simulink model "Boeing787_NewMission_ElectricalThermal_2013"  (R2013a)
settings: Solver=ode23tb  SolverMode=SingleTasking  StartTime=0.0  StopTime=18000  RelTol=1e-3
InitFcn:
  | load('SampleOutput.mat')
  | 
  | load('SampleFuelBurn.mat')
StartFcn:
  | tic
StopFcn:
  | ttt = toc
  | tend = eval(get_param(bdroot,'StopTime'));
  | disp(['Total Simulation Time (s) = ' num2str(ttt) 's']);
  | RTR =  ttt/tend
  | disp(['Simulation Speed is ' num2str(tend/ttt) 'x faster than real-time']);
values from neighbouring files (symbols this model uses):
  CurrentMission = Mission(i)    [mission_plan.m]
  seed = 1    [mission_plan.m]
undefined symbols (not defined in the file or in its folder): FuelBurn
libraries: PowerFlowLib x17, simulink x12, powerlib_meascontrol x1
(part 14 of 17)

== system Boeing787_NewMission_ElectricalThermal_2013/Eng2/Gearbox ==
  w_engine : Inport
  T_gen : Inport  Port=2
  1-tran_efficiency : Gain  Gain=1-Gear_Efficiency/100  SaturateOnIntegerOverflow=on  OutDataTypeStr=Inherit: Same as input  ParamDataTypeStr=Inherit: Same as input
  Gain : Gain  Gain=Gear_Ratio
  Gain1 : Gain  Gain=Gear_Ratio
  Memory1 : Memory
  Sum : Sum  Inputs=-++  SaturateOnIntegerOverflow=on  InputSameDT=on  OutDataTypeStr=Inherit: Same as first input
  gear1 NL loss : Lookup  InputValues=[0;1000;2000;3000;4000;5000;6000]*2*pi/60  Table=[0;0.735;1.334;1.491;1.525;1.212;1.276]  SaturateOnIntegerOverflow=on
  tran_efficiency : Gain  Gain=Gear_Efficiency/4/100  SaturateOnIntegerOverflow=on  OutDataTypeStr=Inherit: Same as input  ParamDataTypeStr=Inherit: Same as input
  w_shaft : Outport
  T_shaft : Outport  Port=2
  wires:
  Sum/1 -> T_shaft/1
  tran_efficiency/1 -> Sum/1
  1-tran_efficiency/1 -> Sum/2
  Memory1/1 -> Sum/3
  gear1 NL loss/1 -> tran_efficiency/1
  w_engine/1 -> gear1 NL loss/1, Gain/1
  T_gen/1 -> 1-tran_efficiency/1, Gain1/1
  Gain1/1 -> Memory1/1
  Gain/1 -> w_shaft/1

== system Boeing787_NewMission_ElectricalThermal_2013/Eng2/Unit Conversion  ==
  Signal_in : Inport
  conv_fcn : Fcn  Expr=u(1)/745.69987
  Converted Signal Out : Outport
  wires:
  conv_fcn/1 -> Converted Signal Out/1
  Signal_in/1 -> conv_fcn/1

== system Boeing787_NewMission_ElectricalThermal_2013/Eng2/Unit Conversion 1 ==
  Signal_in : Inport
  conv_fcn : Fcn  Expr=u(1)/1.8
  Converted Signal Out : Outport
  wires:
  Signal_in/1 -> conv_fcn/1
  conv_fcn/1 -> Converted Signal Out/1

== system Boeing787_NewMission_ElectricalThermal_2013/Eng2/Unit Conversion 4 ==
  Signal_in : Inport
  conv_fcn : Fcn  Expr=u(1)/(1.450377e-1)
  Converted Signal Out : Outport
  wires:
  conv_fcn/1 -> Converted Signal Out/1
  Signal_in/1 -> conv_fcn/1

== system Boeing787_NewMission_ElectricalThermal_2013/Eng2/Unit Conversion 5 ==
  Signal_in : Inport
  conv_fcn : Fcn  Expr=u(1)*.45359237
  Converted Signal Out : Outport
  wires:
  conv_fcn/1 -> Converted Signal Out/1
  Signal_in/1 -> conv_fcn/1

== system Boeing787_NewMission_ElectricalThermal_2013/Electrical/Auto Transformer/Control ==
  Vout : Inport
  ref : Inport  Port=2
  Clock : Clock
  Constant2 : Constant  Value=0
  Integrator : Integrator  ExternalReset=rising
  MinMax : MinMax  Function=max
  Reset on controller start : Step  Time=75  SampleTime=0
  Sum : Sum  Inputs=|-+
  Switch : Switch  Criteria=u2 > Threshold  Threshold=75
  u : Outport
  wires:
  Integrator/1 -> Switch/1
  Vout/1 -> MinMax/1
  Reset on controller start/1 -> Integrator/2
  Switch/1 -> u/1
  Constant2/1 -> Switch/3
  Clock/1 -> Switch/2
  ref/1 -> Sum/2
  Sum/1 -> Integrator/1
  MinMax/1 -> Sum/1

== system Boeing787_NewMission_ElectricalThermal_2013/Electrical/Auto Transformer/Transformer1 ==
  Vin : Inport
  Iout : Inport  Port=2
  u : Inport  Port=3
  Constant : Constant  Value=N2/N1
  Constant1 : Constant  Value=N2/N1
  Gain2 : Gain  Gain=Rp
  Gain3 : Gain  Gain=Rs
  Product : Product  Inputs=3
  Product1 : Product  Inputs=3
  Sum1 : Sum  Inputs=|+-
  Sum2 : Sum  Inputs=|+-
  Vout : Outport
  Iin : Outport  Port=2
  wires:
  Iout/1 -> Product1/3, Gain3/1
  Vin/1 -> Sum1/1
  Gain2/1 -> Sum1/2
  Sum1/1 -> Product/2
  Sum2/1 -> Vout/1
  Gain3/1 -> Sum2/2
  u/1 -> Product1/1, Product/1
  Product/1 -> Sum2/1
  Constant/1 -> Product/3
  Constant1/1 -> Product1/2
  Product1/1 -> Gain2/1, Iin/1

== system Boeing787_NewMission_ElectricalThermal_2013/Electrical/Enabled_AC_Loadloss/Enabled Subsystem ==
  "Vdq0 " : Inport
  CURRENT BASED LOADS : Subsystem
  IMPEDANCE BASED LOADS : Subsystem
  POWER BASED LOADS : Subsystem
  Sum of Elements : Sum  Inputs=+++
  Idq0 : Outport
  loss : Outport  Port=2
  wires:
  POWER BASED LOADS/2(loss) -> loss/1
  IMPEDANCE BASED LOADS/1(Idq0) -> Sum of Elements/3
  Sum of Elements/1 -> Idq0/1
  CURRENT BASED LOADS/1(Idqo) -> Sum of Elements/2
  POWER BASED LOADS/1(Idq0) -> Sum of Elements/1
  "Vdq0 "/1 -> POWER BASED LOADS/1(Vdq0), IMPEDANCE BASED LOADS/1(Vdq0)

== system Boeing787_NewMission_ElectricalThermal_2013/Electrical/Enabled_AC_Loadloss/Enabled Subsystem1 ==
  "Vdq0 " : Inport
  Ext vector : Inport  Port=2
  CURRENT BASED LOADS : Subsystem
  Demux : Demux  Outputs=3
  POWER BASED LOADS : Subsystem
  Sum of Elements : Sum
  Idq0 : Outport
  wires:
  Demux/3 -> CURRENT BASED LOADS/1(Iconst RMS)
  Demux/2 -> POWER BASED LOADS/3(Q)
  Demux/1 -> POWER BASED LOADS/2(P)
  "Vdq0 "/1 -> POWER BASED LOADS/1(Vdq0)
  Ext vector/1 -> Demux/1
  Sum of Elements/1 -> Idq0/1
  POWER BASED LOADS/1(Idq0) -> Sum of Elements/1
  CURRENT BASED LOADS/1(Idqo) -> Sum of Elements/2

== system Boeing787_NewMission_ElectricalThermal_2013/Electrical/Enabled_AC_Loadloss1/Enabled Subsystem ==
  "Vdq0 " : Inport
  CURRENT BASED LOADS : Subsystem
  IMPEDANCE BASED LOADS : Subsystem
  POWER BASED LOADS : Subsystem
  Sum of Elements : Sum  Inputs=+++
  Idq0 : Outport
  loss : Outport  Port=2
  wires:
  POWER BASED LOADS/2(loss) -> loss/1
  IMPEDANCE BASED LOADS/1(Idq0) -> Sum of Elements/3
  CURRENT BASED LOADS/1(Idqo) -> Sum of Elements/2
  POWER BASED LOADS/1(Idq0) -> Sum of Elements/1
  "Vdq0 "/1 -> POWER BASED LOADS/1(Vdq0), IMPEDANCE BASED LOADS/1(Vdq0)
  Sum of Elements/1 -> Idq0/1

== system Boeing787_NewMission_ElectricalThermal_2013/Electrical/Enabled_AC_Loadloss1/Enabled Subsystem1 ==
  "Vdq0 " : Inport
  Ext vector : Inport  Port=2
  CURRENT BASED LOADS : Subsystem
  Demux : Demux  Outputs=3
  POWER BASED LOADS : Subsystem
  Sum of Elements : Sum
  Idq0 : Outport
  wires:
  Demux/3 -> CURRENT BASED LOADS/1(Iconst RMS)
  Demux/2 -> POWER BASED LOADS/3(Q)
  Demux/1 -> POWER BASED LOADS/2(P)
  "Vdq0 "/1 -> POWER BASED LOADS/1(Vdq0)
  Ext vector/1 -> Demux/1
  Sum of Elements/1 -> Idq0/1
  POWER BASED LOADS/1(Idq0) -> Sum of Elements/1
  CURRENT BASED LOADS/1(Idqo) -> Sum of Elements/2

== system Boeing787_NewMission_ElectricalThermal_2013/Electrical/Generation Unit Sync-Sync/Chopper (Averaged) ==
  vin : Inport
  q : Inport  Port=2
  Temperature : Inport  Port=3
  1/R : Gain  Gain=1/(R_fd_exc*VBFD_exc/IBFD_exc)/100/2*3/100  SaturateOnIntegerOverflow=on  OutDataTypeStr=Inherit: Same as input  ParamDataTypeStr=Inherit: Same as input
  Divide : Product  Inputs=*/
  Dot Product : DotProduct  InputSameDT=on  OutDataTypeStr=Inherit: Inherit via internal rule
  Dot Product1 : DotProduct  InputSameDT=on  OutDataTypeStr=Inherit: Inherit via internal rule
  Gain2 : Gain  Gain=1000*2/3
  Saturation : Saturate  UpperLimit=1  LowerLimit=0
  iout : Outport
  iin : Outport  Port=2
  wires:
  Divide/1 -> Gain2/1
  Temperature/1 -> Divide/2
  1/R/1 -> Divide/1
  Gain2/1 -> iout/1, Dot Product1/1
  vin/1 -> Dot Product/1
  q/1 -> Saturation/1
  Dot Product/1 -> 1/R/1
  Saturation/1 -> Dot Product/2, Dot Product1/2
  Dot Product1/1 -> iin/1

== system Boeing787_NewMission_ElectricalThermal_2013/Electrical/Generation Unit Sync-Sync/Exciter ==
  note: Dynamic model of P.U. Synchronous Generators v1.0
      | Base frequency is 60 Hz
      | Network transients are omitted
      | by Tutku Buyukdegirmenci
  note: Core Dynaimcs
  note: Outputs
  note: Inputs
  note: 0 axis to be implemented
  idq0 : Inport
  w : Inport  Port=2
  ifd' : Inport  Port=3
  Temp : Inport  Port=4
  Demux : Demux  Outputs=3
  Divide : Product  Inputs=*/
  Dynamics : Subsystem
  Electromagnetic Torque Output Power : Subsystem
  Gain1 : Gain  Gain=Xmd_exc/R_fd_exc/VBFD_exc
  Gain2 : Gain  Gain=1/wB_exc
  Gain3 : Gain  Gain=R_fd_exc*VBFD_exc/IBFD_exc
  Gain4 : Gain  Gain=P_exc/2
  Generator Power Loss : Subsystem
  Mux : Mux  Inputs=3
  Product : Product
  Stator Voltage : Subsystem
  Terminator2 : Terminator
  Terminator3 : Terminator
  Terminator4 : Terminator
  V0 : Constant  Value=0
  p.u. transform currents : Gain  Gain=-1/IBDQ_exc
  p.u. transform torque : Gain  Gain=TB_exc
  p.u. transform voltages : Gain  Gain=VBDQ_exc
  vdq0 : Outport
  Te : Outport  Port=2
  vfd' : Outport  Port=3
  Ploss : Outport  Port=4
  wires:
  [R_temp_delta] -> Divide/2, Product/2
  Product/1 -> Gain1/1, vfd'/1
  Divide/1 -> [Efd]
  Gain1/1 -> Divide/1
  Gain3/1 -> Product/1  "vfd'"
  [R_temp_delta] -> Dynamics/4(Temp), Stator Voltage/8(Temp)
  Temp/1 -> [R_temp_delta]
  Gain4/1 -> Gain2/1
  [Efd] -> Dynamics/3(Efd)
  ifd'/1 -> Gain3/1
  idq0/1 -> p.u. transform currents/1
  p.u. transform voltages/1 -> vdq0/1
  Generator Power Loss/3(PLOSS) -> Terminator4/1, Ploss/1
  Generator Power Loss/2(PM) -> Terminator3/1
  Generator Power Loss/1(PE) -> Terminator2/1
  [Te] -> Generator Power Loss/5(Te)
  [nu] -> Generator Power Loss/6(w/ws)
  [Iq] -> Generator Power Loss/4(Iq)
  [Id] -> Generator Power Loss/3(Id)
  [Vq] -> Generator Power Loss/2(Eq)
  [Vd] -> Generator Power Loss/1(Ed)
  p.u. transform torque/1 -> Te/1
  p.u. transform currents/1 -> Demux/1
  [Te] -> p.u. transform torque/1
  Electromagnetic Torque Output Power/1(TE) -> [Te]
  [nu] -> Stator Voltage/7(w/ws)
  V0/1 -> Mux/3
  [Vq] -> Mux/2
  [Vd] -> Mux/1
  Mux/1 -> p.u. transform voltages/1
  [Iq] -> Electromagnetic Torque Output Power/2(Iq), Stator Voltage/2(Iq)
  [Id] -> Electromagnetic Torque Output Power/1(Id), Stator Voltage/1(Id)
  [Iq] -> Dynamics/2(Iq)
  [Id] -> Dynamics/1(Id)
  Gain2/1 -> [nu]
  Demux/2 -> [Iq]
  Demux/1 -> [Id]
  w/1 -> Gain4/1
  Stator Voltage/1(Ed) -> [Vd]
  Stator Voltage/2(Eq) -> [Vq]
  Dynamics/4(Phi_2q) -> Electromagnetic Torque Output Power/6(Phi_2q), Stator Voltage/6(Phi_2q)
  Dynamics/3(Phi_1d) -> Electromagnetic Torque Output Power/5(Phi_1d), Stator Voltage/5(Phi_1d)
  Dynamics/2(Ed1) -> Electromagnetic Torque Output Power/4(Ed1), Stator Voltage/4(Ed1)
  Dynamics/1(Eq1) -> Electromagnetic Torque Output Power/3(Eq1), Stator Voltage/3(Eq1)

== system Boeing787_NewMission_ElectricalThermal_2013/Electrical/Generation Unit Sync-Sync/Generator ==
  note: 0 axis to be implemented
  note: Inputs
  note: Outputs
  note: Core Dynaimcs
  note: Dynamic model of P.U. Synchronous Generators v1.0
      | Base frequency is 60 Hz
      | Network transients are omitted
      | by Tutku Buyukdegirmenci
  idq0 : Inport
  w : Inport  Port=2
  ifd' : Inport  Port=3
  Temp : Inport  Port=4
  Demux : Demux  Outputs=3
  Divide : Product  Inputs=*/
  Dynamics : Subsystem
  Electromagnetic Torque Output Power : Subsystem
  Gain1 : Gain  Gain=Xmd/R_fd/VBFD
  Gain2 : Gain  Gain=1/wB
  Gain3 : Gain  Gain=R_fd*VBFD/IBFD
  Gain4 : Gain  Gain=P/2
  Generator Power Loss : Subsystem
  Mux : Mux  Inputs=3
  Product : Product
  Stator Voltage : Subsystem
  Terminator2 : Terminator
  Terminator3 : Terminator
  Terminator4 : Terminator
  V0 : Constant  Value=0
  p.u. transform currents : Gain  Gain=-1/IBDQ
  p.u. transform torque : Gain  Gain=TB
  p.u. transform voltages : Gain  Gain=VBDQ
  vdq0 : Outport
  Te : Outport  Port=2
  vfd' : Outport  Port=3
  Ploss : Outport  Port=4
  wires:
  [R_temp_delta] -> Dynamics/4(Temp), Stator Voltage/8(Temp)
  [R_temp_delta] -> Product/2, Divide/2
  Product/1 -> vfd'/1, Gain1/1
  Gain3/1 -> Product/1  "vfd'"
  Divide/1 -> [Efd]
  Gain1/1 -> Divide/1
  Temp/1 -> [R_temp_delta]
  Dynamics/1(Eq1) -> Stator Voltage/3(Eq1), Electromagnetic Torque Output Power/3(Eq1)
  Dynamics/2(Ed1) -> Stator Voltage/4(Ed1), Electromagnetic Torque Output Power/4(Ed1)
  Dynamics/3(Phi_1d) -> Stator Voltage/5(Phi_1d), Electromagnetic Torque Output Power/5(Phi_1d)
  Dynamics/4(Phi_2q) -> Stator Voltage/6(Phi_2q), Electromagnetic Torque Output Power/6(Phi_2q)
  Stator Voltage/2(Eq) -> [Vq]
  Stator Voltage/1(Ed) -> [Vd]
  w/1 -> Gain4/1
  Demux/1 -> [Id]
  Demux/2 -> [Iq]
  Gain2/1 -> [nu]
  [Id] -> Dynamics/1(Id)
  [Iq] -> Dynamics/2(Iq)
  [Id] -> Stator Voltage/1(Id), Electromagnetic Torque Output Power/1(Id)
  [Iq] -> Stator Voltage/2(Iq), Electromagnetic Torque Output Power/2(Iq)
  Mux/1 -> p.u. transform voltages/1
  [Vd] -> Mux/1
  [Vq] -> Mux/2
  V0/1 -> Mux/3
  [nu] -> Stator Voltage/7(w/ws)
  Electromagnetic Torque Output Power/1(TE) -> [Te]
  [Te] -> p.u. transform torque/1
  p.u. transform currents/1 -> Demux/1
  p.u. transform torque/1 -> Te/1
  [Vd] -> Generator Power Loss/1(Ed)
  [Vq] -> Generator Power Loss/2(Eq)
  [Id] -> Generator Power Loss/3(Id)
  [Iq] -> Generator Power Loss/4(Iq)
  [nu] -> Generator Power Loss/6(w/ws)
  [Te] -> Generator Power Loss/5(Te)
  Generator Power Loss/1(PE) -> Terminator2/1
  Generator Power Loss/2(PM) -> Terminator3/1
  Generator Power Loss/3(PLOSS) -> Terminator4/1, Ploss/1
  p.u. transform voltages/1 -> vdq0/1
  idq0/1 -> p.u. transform currents/1
  ifd'/1 -> Gain3/1
  [Efd] -> Dynamics/3(Efd)
  Gain4/1 -> Gain2/1

== system Boeing787_NewMission_ElectricalThermal_2013/Electrical/Generation Unit Sync-Sync1/Chopper (Averaged) ==
  vin : Inport
  q : Inport  Port=2
  Temperature : Inport  Port=3
  1/R : Gain  Gain=1/(R_fd_exc*VBFD_exc/IBFD_exc)/100/2*3/100  SaturateOnIntegerOverflow=on  OutDataTypeStr=Inherit: Same as input  ParamDataTypeStr=Inherit: Same as input
  Divide : Product  Inputs=*/
  Dot Product : DotProduct  InputSameDT=on  OutDataTypeStr=Inherit: Inherit via internal rule
  Dot Product1 : DotProduct  InputSameDT=on  OutDataTypeStr=Inherit: Inherit via internal rule
  Gain2 : Gain  Gain=1000*2/3
  Saturation : Saturate  UpperLimit=1  LowerLimit=0
  iout : Outport
  iin : Outport  Port=2
  wires:
  Dot Product1/1 -> iin/1
  Saturation/1 -> Dot Product1/2, Dot Product/2
  Dot Product/1 -> 1/R/1
  q/1 -> Saturation/1
  vin/1 -> Dot Product/1
  Gain2/1 -> Dot Product1/1, iout/1
  1/R/1 -> Divide/1
  Temperature/1 -> Divide/2
  Divide/1 -> Gain2/1

== system Boeing787_NewMission_ElectricalThermal_2013/Electrical/Generation Unit Sync-Sync1/Exciter ==
  note: 0 axis to be implemented
  note: Inputs
  note: Outputs
  note: Core Dynaimcs
  note: Dynamic model of P.U. Synchronous Generators v1.0
      | Base frequency is 60 Hz
      | Network transients are omitted
      | by Tutku Buyukdegirmenci
  idq0 : Inport
  w : Inport  Port=2
  ifd' : Inport  Port=3
  Temp : Inport  Port=4
  Demux : Demux  Outputs=3
  Divide : Product  Inputs=*/
  Dynamics : Subsystem
  Electromagnetic Torque Output Power : Subsystem
  Gain1 : Gain  Gain=Xmd_exc/R_fd_exc/VBFD_exc
  Gain2 : Gain  Gain=1/wB_exc
  Gain3 : Gain  Gain=R_fd_exc*VBFD_exc/IBFD_exc
  Gain4 : Gain  Gain=P_exc/2
  Generator Power Loss : Subsystem
  Mux : Mux  Inputs=3
  Product : Product
  Stator Voltage : Subsystem
  Terminator2 : Terminator
  Terminator3 : Terminator
  Terminator4 : Terminator
  V0 : Constant  Value=0
  p.u. transform currents : Gain  Gain=-1/IBDQ_exc
  p.u. transform torque : Gain  Gain=TB_exc
  p.u. transform voltages : Gain  Gain=VBDQ_exc
  vdq0 : Outport
  Te : Outport  Port=2
  vfd' : Outport  Port=3
  Ploss : Outport  Port=4
  wires:
  Dynamics/1(Eq1) -> Stator Voltage/3(Eq1), Electromagnetic Torque Output Power/3(Eq1)
  Dynamics/2(Ed1) -> Stator Voltage/4(Ed1), Electromagnetic Torque Output Power/4(Ed1)
  Dynamics/3(Phi_1d) -> Stator Voltage/5(Phi_1d), Electromagnetic Torque Output Power/5(Phi_1d)
  Dynamics/4(Phi_2q) -> Stator Voltage/6(Phi_2q), Electromagnetic Torque Output Power/6(Phi_2q)
  Stator Voltage/2(Eq) -> [Vq]
  Stator Voltage/1(Ed) -> [Vd]
  w/1 -> Gain4/1
  Demux/1 -> [Id]
  Demux/2 -> [Iq]
  Gain2/1 -> [nu]
  [Id] -> Dynamics/1(Id)
  [Iq] -> Dynamics/2(Iq)
  [Id] -> Stator Voltage/1(Id), Electromagnetic Torque Output Power/1(Id)
  [Iq] -> Stator Voltage/2(Iq), Electromagnetic Torque Output Power/2(Iq)
  Mux/1 -> p.u. transform voltages/1
  [Vd] -> Mux/1
  [Vq] -> Mux/2
  V0/1 -> Mux/3
  [nu] -> Stator Voltage/7(w/ws)
  Electromagnetic Torque Output Power/1(TE) -> [Te]
  [Te] -> p.u. transform torque/1
  p.u. transform currents/1 -> Demux/1
  p.u. transform torque/1 -> Te/1
  [Vd] -> Generator Power Loss/1(Ed)
  [Vq] -> Generator Power Loss/2(Eq)
  [Id] -> Generator Power Loss/3(Id)
  [Iq] -> Generator Power Loss/4(Iq)
  [nu] -> Generator Power Loss/6(w/ws)
  [Te] -> Generator Power Loss/5(Te)
  Generator Power Loss/1(PE) -> Terminator2/1
  Generator Power Loss/2(PM) -> Terminator3/1
  Generator Power Loss/3(PLOSS) -> Ploss/1, Terminator4/1
  p.u. transform voltages/1 -> vdq0/1
  idq0/1 -> p.u. transform currents/1
  ifd'/1 -> Gain3/1
  [Efd] -> Dynamics/3(Efd)
  Gain4/1 -> Gain2/1
  Temp/1 -> [R_temp_delta]
  [R_temp_delta] -> Stator Voltage/8(Temp), Dynamics/4(Temp)
  Gain3/1 -> Product/1  "vfd'"
  Gain1/1 -> Divide/1
  Divide/1 -> [Efd]
  Product/1 -> vfd'/1, Gain1/1
  [R_temp_delta] -> Product/2, Divide/2

== system Boeing787_NewMission_ElectricalThermal_2013/Electrical/Generation Unit Sync-Sync1/Generator ==
  note: Dynamic model of P.U. Synchronous Generators v1.0
      | Base frequency is 60 Hz
      | Network transients are omitted
      | by Tutku Buyukdegirmenci
  note: Core Dynaimcs
  note: Outputs
  note: Inputs
  note: 0 axis to be implemented
  idq0 : Inport
  w : Inport  Port=2
  ifd' : Inport  Port=3
  Temp : Inport  Port=4
  Demux : Demux  Outputs=3
  Divide : Product  Inputs=*/
  Dynamics : Subsystem
  Electromagnetic Torque Output Power : Subsystem
  Gain1 : Gain  Gain=Xmd/R_fd/VBFD
  Gain2 : Gain  Gain=1/wB
  Gain3 : Gain  Gain=R_fd*VBFD/IBFD
  Gain4 : Gain  Gain=P/2
  Generator Power Loss : Subsystem
  Mux : Mux  Inputs=3
  Product : Product
  Stator Voltage : Subsystem
  Terminator2 : Terminator
  Terminator3 : Terminator
  Terminator4 : Terminator
  V0 : Constant  Value=0
  p.u. transform currents : Gain  Gain=-1/IBDQ
  p.u. transform torque : Gain  Gain=TB
  p.u. transform voltages : Gain  Gain=VBDQ
  vdq0 : Outport
  Te : Outport  Port=2
  vfd' : Outport  Port=3
  Ploss : Outport  Port=4
  wires:
  Gain4/1 -> Gain2/1
  [Efd] -> Dynamics/3(Efd)
  ifd'/1 -> Gain3/1
  idq0/1 -> p.u. transform currents/1
  p.u. transform voltages/1 -> vdq0/1
  Generator Power Loss/3(PLOSS) -> Ploss/1, Terminator4/1
  Generator Power Loss/2(PM) -> Terminator3/1
  Generator Power Loss/1(PE) -> Terminator2/1
  [Te] -> Generator Power Loss/5(Te)
  [nu] -> Generator Power Loss/6(w/ws)
  [Iq] -> Generator Power Loss/4(Iq)
  [Id] -> Generator Power Loss/3(Id)
  [Vq] -> Generator Power Loss/2(Eq)
  [Vd] -> Generator Power Loss/1(Ed)
  p.u. transform torque/1 -> Te/1
  p.u. transform currents/1 -> Demux/1
  [Te] -> p.u. transform torque/1
  Electromagnetic Torque Output Power/1(TE) -> [Te]
  [nu] -> Stator Voltage/7(w/ws)
  V0/1 -> Mux/3
  [Vq] -> Mux/2
  [Vd] -> Mux/1
  Mux/1 -> p.u. transform voltages/1
  [Iq] -> Electromagnetic Torque Output Power/2(Iq), Stator Voltage/2(Iq)
  [Id] -> Electromagnetic Torque Output Power/1(Id), Stator Voltage/1(Id)
  [Iq] -> Dynamics/2(Iq)
  [Id] -> Dynamics/1(Id)
  Gain2/1 -> [nu]
  Demux/2 -> [Iq]
  Demux/1 -> [Id]
  w/1 -> Gain4/1
  Stator Voltage/1(Ed) -> [Vd]
  Stator Voltage/2(Eq) -> [Vq]
  Dynamics/4(Phi_2q) -> Electromagnetic Torque Output Power/6(Phi_2q), Stator Voltage/6(Phi_2q)
  Dynamics/3(Phi_1d) -> Electromagnetic Torque Output Power/5(Phi_1d), Stator Voltage/5(Phi_1d)
  Dynamics/2(Ed1) -> Electromagnetic Torque Output Power/4(Ed1), Stator Voltage/4(Ed1)
  Dynamics/1(Eq1) -> Electromagnetic Torque Output Power/3(Eq1), Stator Voltage/3(Eq1)
  Temp/1 -> [R_temp_delta]
  Gain1/1 -> Divide/1
  Divide/1 -> [Efd]
  Gain3/1 -> Product/1  "vfd'"
  Product/1 -> Gain1/1, vfd'/1
  [R_temp_delta] -> Divide/2, Product/2
  [R_temp_delta] -> Stator Voltage/8(Temp), Dynamics/4(Temp)

== system Boeing787_NewMission_ElectricalThermal_2013/Electrical/Generation Unit Sync-Sync2/Chopper (Averaged) ==
  vin : Inport
  q : Inport  Port=2
  Temperature : Inport  Port=3
  1/R : Gain  Gain=1/(R_fd_exc*VBFD_exc/IBFD_exc)/100/2*3/100  SaturateOnIntegerOverflow=on  OutDataTypeStr=Inherit: Same as input  ParamDataTypeStr=Inherit: Same as input
  Divide : Product  Inputs=*/
  Dot Product : DotProduct  InputSameDT=on  OutDataTypeStr=Inherit: Inherit via internal rule
  Dot Product1 : DotProduct  InputSameDT=on  OutDataTypeStr=Inherit: Inherit via internal rule
  Gain2 : Gain  Gain=1000*2/3
  Saturation : Saturate  UpperLimit=1  LowerLimit=0
  iout : Outport
  iin : Outport  Port=2
  wires:
  Divide/1 -> Gain2/1
  Temperature/1 -> Divide/2
  1/R/1 -> Divide/1
  Gain2/1 -> iout/1, Dot Product1/1
  vin/1 -> Dot Product/1
  q/1 -> Saturation/1
  Dot Product/1 -> 1/R/1
  Saturation/1 -> Dot Product/2, Dot Product1/2
  Dot Product1/1 -> iin/1

== system Boeing787_NewMission_ElectricalThermal_2013/Electrical/Generation Unit Sync-Sync2/Exciter ==
  note: Dynamic model of P.U. Synchronous Generators v1.0
      | Base frequency is 60 Hz
      | Network transients are omitted
      | by Tutku Buyukdegirmenci
  note: Core Dynaimcs
  note: Outputs
  note: Inputs
  note: 0 axis to be implemented
  idq0 : Inport
  w : Inport  Port=2
  ifd' : Inport  Port=3
  Temp : Inport  Port=4
  Demux : Demux  Outputs=3
  Divide : Product  Inputs=*/
  Dynamics : Subsystem
  Electromagnetic Torque Output Power : Subsystem
  Gain1 : Gain  Gain=Xmd_exc/R_fd_exc/VBFD_exc
  Gain2 : Gain  Gain=1/wB_exc
  Gain3 : Gain  Gain=R_fd_exc*VBFD_exc/IBFD_exc
  Gain4 : Gain  Gain=P_exc/2
  Generator Power Loss : Subsystem
  Mux : Mux  Inputs=3
  Product : Product
  Stator Voltage : Subsystem
  Terminator2 : Terminator
  Terminator3 : Terminator
  Terminator4 : Terminator
  V0 : Constant  Value=0
  p.u. transform currents : Gain  Gain=-1/IBDQ_exc
  p.u. transform torque : Gain  Gain=TB_exc
  p.u. transform voltages : Gain  Gain=VBDQ_exc
  vdq0 : Outport
  Te : Outport  Port=2
  vfd' : Outport  Port=3
  Ploss : Outport  Port=4
  wires:
  [R_temp_delta] -> Divide/2, Product/2
  Product/1 -> Gain1/1, vfd'/1
  Divide/1 -> [Efd]
  Gain1/1 -> Divide/1
  Gain3/1 -> Product/1  "vfd'"
  [R_temp_delta] -> Dynamics/4(Temp), Stator Voltage/8(Temp)
  Temp/1 -> [R_temp_delta]
  Gain4/1 -> Gain2/1
  [Efd] -> Dynamics/3(Efd)
  ifd'/1 -> Gain3/1
  idq0/1 -> p.u. transform currents/1
  p.u. transform voltages/1 -> vdq0/1
  Generator Power Loss/3(PLOSS) -> Terminator4/1, Ploss/1
  Generator Power Loss/2(PM) -> Terminator3/1
  Generator Power Loss/1(PE) -> Terminator2/1
  [Te] -> Generator Power Loss/5(Te)
  [nu] -> Generator Power Loss/6(w/ws)
  [Iq] -> Generator Power Loss/4(Iq)
  [Id] -> Generator Power Loss/3(Id)
  [Vq] -> Generator Power Loss/2(Eq)
  [Vd] -> Generator Power Loss/1(Ed)
  p.u. transform torque/1 -> Te/1
  p.u. transform currents/1 -> Demux/1
  [Te] -> p.u. transform torque/1
  Electromagnetic Torque Output Power/1(TE) -> [Te]
  [nu] -> Stator Voltage/7(w/ws)
  V0/1 -> Mux/3
  [Vq] -> Mux/2
  [Vd] -> Mux/1
  Mux/1 -> p.u. transform voltages/1
  [Iq] -> Electromagnetic Torque Output Power/2(Iq), Stator Voltage/2(Iq)
  [Id] -> Electromagnetic Torque Output Power/1(Id), Stator Voltage/1(Id)
  [Iq] -> Dynamics/2(Iq)
  [Id] -> Dynamics/1(Id)
  Gain2/1 -> [nu]
  Demux/2 -> [Iq]
  Demux/1 -> [Id]
  w/1 -> Gain4/1
  Stator Voltage/1(Ed) -> [Vd]
  Stator Voltage/2(Eq) -> [Vq]
  Dynamics/4(Phi_2q) -> Electromagnetic Torque Output Power/6(Phi_2q), Stator Voltage/6(Phi_2q)
  Dynamics/3(Phi_1d) -> Electromagnetic Torque Output Power/5(Phi_1d), Stator Voltage/5(Phi_1d)
  Dynamics/2(Ed1) -> Electromagnetic Torque Output Power/4(Ed1), Stator Voltage/4(Ed1)
  Dynamics/1(Eq1) -> Electromagnetic Torque Output Power/3(Eq1), Stator Voltage/3(Eq1)

== system Boeing787_NewMission_ElectricalThermal_2013/Electrical/Generation Unit Sync-Sync2/Generator ==
  note: 0 axis to be implemented
  note: Inputs
  note: Outputs
  note: Core Dynaimcs
  note: Dynamic model of P.U. Synchronous Generators v1.0
      | Base frequency is 60 Hz
      | Network transients are omitted
      | by Tutku Buyukdegirmenci
  idq0 : Inport
  w : Inport  Port=2
  ifd' : Inport  Port=3
  Temp : Inport  Port=4
  Demux : Demux  Outputs=3
  Divide : Product  Inputs=*/
  Dynamics : Subsystem
  Electromagnetic Torque Output Power : Subsystem
  Gain1 : Gain  Gain=Xmd/R_fd/VBFD
  Gain2 : Gain  Gain=1/wB
  Gain3 : Gain  Gain=R_fd*VBFD/IBFD
  Gain4 : Gain  Gain=P/2
  Generator Power Loss : Subsystem
  Mux : Mux  Inputs=3
  Product : Product
  Stator Voltage : Subsystem
  Terminator2 : Terminator
  Terminator3 : Terminator
  Terminator4 : Terminator
  V0 : Constant  Value=0
  p.u. transform currents : Gain  Gain=-1/IBDQ
  p.u. transform torque : Gain  Gain=TB
  p.u. transform voltages : Gain  Gain=VBDQ
  vdq0 : Outport
  Te : Outport  Port=2
  vfd' : Outport  Port=3
  Ploss : Outport  Port=4
  wires:
  [R_temp_delta] -> Dynamics/4(Temp), Stator Voltage/8(Temp)
  [R_temp_delta] -> Product/2, Divide/2
  Product/1 -> vfd'/1, Gain1/1
  Gain3/1 -> Product/1  "vfd'"
  Divide/1 -> [Efd]
  Gain1/1 -> Divide/1
  Temp/1 -> [R_temp_delta]
  Dynamics/1(Eq1) -> Stator Voltage/3(Eq1), Electromagnetic Torque Output Power/3(Eq1)
  Dynamics/2(Ed1) -> Stator Voltage/4(Ed1), Electromagnetic Torque Output Power/4(Ed1)
  Dynamics/3(Phi_1d) -> Stator Voltage/5(Phi_1d), Electromagnetic Torque Output Power/5(Phi_1d)
  Dynamics/4(Phi_2q) -> Stator Voltage/6(Phi_2q), Electromagnetic Torque Output Power/6(Phi_2q)
  Stator Voltage/2(Eq) -> [Vq]
  Stator Voltage/1(Ed) -> [Vd]
  w/1 -> Gain4/1
  Demux/1 -> [Id]
  Demux/2 -> [Iq]
  Gain2/1 -> [nu]
  [Id] -> Dynamics/1(Id)
  [Iq] -> Dynamics/2(Iq)
  [Id] -> Stator Voltage/1(Id), Electromagnetic Torque Output Power/1(Id)
  [Iq] -> Stator Voltage/2(Iq), Electromagnetic Torque Output Power/2(Iq)
  Mux/1 -> p.u. transform voltages/1
  [Vd] -> Mux/1
  [Vq] -> Mux/2
  V0/1 -> Mux/3
  [nu] -> Stator Voltage/7(w/ws)
  Electromagnetic Torque Output Power/1(TE) -> [Te]
  [Te] -> p.u. transform torque/1
  p.u. transform currents/1 -> Demux/1
  p.u. transform torque/1 -> Te/1
  [Vd] -> Generator Power Loss/1(Ed)
  [Vq] -> Generator Power Loss/2(Eq)
  [Id] -> Generator Power Loss/3(Id)
  [Iq] -> Generator Power Loss/4(Iq)
  [nu] -> Generator Power Loss/6(w/ws)
  [Te] -> Generator Power Loss/5(Te)
  Generator Power Loss/1(PE) -> Terminator2/1
  Generator Power Loss/2(PM) -> Terminator3/1
  Generator Power Loss/3(PLOSS) -> Terminator4/1, Ploss/1
  p.u. transform voltages/1 -> vdq0/1
  idq0/1 -> p.u. transform currents/1
  ifd'/1 -> Gain3/1
  [Efd] -> Dynamics/3(Efd)
  Gain4/1 -> Gain2/1

== system Boeing787_NewMission_ElectricalThermal_2013/Electrical/Generation Unit Sync-Sync3/Chopper (Averaged) ==
  vin : Inport
  q : Inport  Port=2
  Temperature : Inport  Port=3
  1/R : Gain  Gain=1/(R_fd_exc*VBFD_exc/IBFD_exc)/100/2*3/100  SaturateOnIntegerOverflow=on  OutDataTypeStr=Inherit: Same as input  ParamDataTypeStr=Inherit: Same as input
  Divide : Product  Inputs=*/
  Dot Product : DotProduct  InputSameDT=on  OutDataTypeStr=Inherit: Inherit via internal rule
  Dot Product1 : DotProduct  InputSameDT=on  OutDataTypeStr=Inherit: Inherit via internal rule
  Gain2 : Gain  Gain=1000*2/3
  Saturation : Saturate  UpperLimit=1  LowerLimit=0
  iout : Outport
  iin : Outport  Port=2
  wires:
  Dot Product1/1 -> iin/1
  Saturation/1 -> Dot Product1/2, Dot Product/2
  Dot Product/1 -> 1/R/1
  q/1 -> Saturation/1
  vin/1 -> Dot Product/1
  Gain2/1 -> Dot Product1/1, iout/1
  1/R/1 -> Divide/1
  Temperature/1 -> Divide/2
  Divide/1 -> Gain2/1

== system Boeing787_NewMission_ElectricalThermal_2013/Electrical/Generation Unit Sync-Sync3/Exciter ==
  note: 0 axis to be implemented
  note: Inputs
  note: Outputs
  note: Core Dynaimcs
  note: Dynamic model of P.U. Synchronous Generators v1.0
      | Base frequency is 60 Hz
      | Network transients are omitted
      | by Tutku Buyukdegirmenci
  idq0 : Inport
  w : Inport  Port=2
  ifd' : Inport  Port=3
  Temp : Inport  Port=4
  Demux : Demux  Outputs=3
  Divide : Product  Inputs=*/
  Dynamics : Subsystem
  Electromagnetic Torque Output Power : Subsystem
  Gain1 : Gain  Gain=Xmd_exc/R_fd_exc/VBFD_exc
  Gain2 : Gain  Gain=1/wB_exc
  Gain3 : Gain  Gain=R_fd_exc*VBFD_exc/IBFD_exc
  Gain4 : Gain  Gain=P_exc/2
  Generator Power Loss : Subsystem
  Mux : Mux  Inputs=3
  Product : Product
  Stator Voltage : Subsystem
  Terminator2 : Terminator
  Terminator3 : Terminator
  Terminator4 : Terminator
  V0 : Constant  Value=0
  p.u. transform currents : Gain  Gain=-1/IBDQ_exc
  p.u. transform torque : Gain  Gain=TB_exc
  p.u. transform voltages : Gain  Gain=VBDQ_exc
  vdq0 : Outport
  Te : Outport  Port=2
  vfd' : Outport  Port=3
  Ploss : Outport  Port=4
  wires:
  Dynamics/1(Eq1) -> Stator Voltage/3(Eq1), Electromagnetic Torque Output Power/3(Eq1)
  Dynamics/2(Ed1) -> Stator Voltage/4(Ed1), Electromagnetic Torque Output Power/4(Ed1)
  Dynamics/3(Phi_1d) -> Stator Voltage/5(Phi_1d), Electromagnetic Torque Output Power/5(Phi_1d)
  Dynamics/4(Phi_2q) -> Stator Voltage/6(Phi_2q), Electromagnetic Torque Output Power/6(Phi_2q)
  Stator Voltage/2(Eq) -> [Vq]
  Stator Voltage/1(Ed) -> [Vd]
  w/1 -> Gain4/1
  Demux/1 -> [Id]
  Demux/2 -> [Iq]
  Gain2/1 -> [nu]
  [Id] -> Dynamics/1(Id)
  [Iq] -> Dynamics/2(Iq)
  [Id] -> Stator Voltage/1(Id), Electromagnetic Torque Output Power/1(Id)
  [Iq] -> Stator Voltage/2(Iq), Electromagnetic Torque Output Power/2(Iq)
  Mux/1 -> p.u. transform voltages/1
  [Vd] -> Mux/1
  [Vq] -> Mux/2
  V0/1 -> Mux/3
  [nu] -> Stator Voltage/7(w/ws)
  Electromagnetic Torque Output Power/1(TE) -> [Te]
  [Te] -> p.u. transform torque/1
  p.u. transform currents/1 -> Demux/1
  p.u. transform torque/1 -> Te/1
  [Vd] -> Generator Power Loss/1(Ed)
  [Vq] -> Generator Power Loss/2(Eq)
  [Id] -> Generator Power Loss/3(Id)
  [Iq] -> Generator Power Loss/4(Iq)
  [nu] -> Generator Power Loss/6(w/ws)
  [Te] -> Generator Power Loss/5(Te)
  Generator Power Loss/1(PE) -> Terminator2/1
  Generator Power Loss/2(PM) -> Terminator3/1
  Generator Power Loss/3(PLOSS) -> Ploss/1, Terminator4/1
  p.u. transform voltages/1 -> vdq0/1
  idq0/1 -> p.u. transform currents/1
  ifd'/1 -> Gain3/1
  [Efd] -> Dynamics/3(Efd)
  Gain4/1 -> Gain2/1
  Temp/1 -> [R_temp_delta]
  [R_temp_delta] -> Stator Voltage/8(Temp), Dynamics/4(Temp)
  Gain3/1 -> Product/1  "vfd'"
  Gain1/1 -> Divide/1
  Divide/1 -> [Efd]
  Product/1 -> vfd'/1, Gain1/1
  [R_temp_delta] -> Product/2, Divide/2

== system Boeing787_NewMission_ElectricalThermal_2013/Electrical/Generation Unit Sync-Sync3/Generator ==
  note: Dynamic model of P.U. Synchronous Generators v1.0
      | Base frequency is 60 Hz
      | Network transients are omitted
      | by Tutku Buyukdegirmenci
  note: Core Dynaimcs
  note: Outputs
  note: Inputs
  note: 0 axis to be implemented
  idq0 : Inport
  w : Inport  Port=2
  ifd' : Inport  Port=3
  Temp : Inport  Port=4
  Demux : Demux  Outputs=3
  Divide : Product  Inputs=*/
  Dynamics : Subsystem
  Electromagnetic Torque Output Power : Subsystem
  Gain1 : Gain  Gain=Xmd/R_fd/VBFD
  Gain2 : Gain  Gain=1/wB
  Gain3 : Gain  Gain=R_fd*VBFD/IBFD
  Gain4 : Gain  Gain=P/2
  Generator Power Loss : Subsystem
  Mux : Mux  Inputs=3
  Product : Product
  Stator Voltage : Subsystem
  Terminator2 : Terminator
  Terminator3 : Terminator
  Terminator4 : Terminator
  V0 : Constant  Value=0
  p.u. transform currents : Gain  Gain=-1/IBDQ
  p.u. transform torque : Gain  Gain=TB
  p.u. transform voltages : Gain  Gain=VBDQ
  vdq0 : Outport
  Te : Outport  Port=2
  vfd' : Outport  Port=3
  Ploss : Outport  Port=4
  wires:
  Gain4/1 -> Gain2/1
  [Efd] -> Dynamics/3(Efd)
  ifd'/1 -> Gain3/1
  idq0/1 -> p.u. transform currents/1
  p.u. transform voltages/1 -> vdq0/1
  Generator Power Loss/3(PLOSS) -> Ploss/1, Terminator4/1
  Generator Power Loss/2(PM) -> Terminator3/1
  Generator Power Loss/1(PE) -> Terminator2/1
  [Te] -> Generator Power Loss/5(Te)
  [nu] -> Generator Power Loss/6(w/ws)
  [Iq] -> Generator Power Loss/4(Iq)
  [Id] -> Generator Power Loss/3(Id)
  [Vq] -> Generator Power Loss/2(Eq)
  [Vd] -> Generator Power Loss/1(Ed)
  p.u. transform torque/1 -> Te/1
  p.u. transform currents/1 -> Demux/1
  [Te] -> p.u. transform torque/1
  Electromagnetic Torque Output Power/1(TE) -> [Te]
  [nu] -> Stator Voltage/7(w/ws)
  V0/1 -> Mux/3
  [Vq] -> Mux/2
  [Vd] -> Mux/1
  Mux/1 -> p.u. transform voltages/1
  [Iq] -> Electromagnetic Torque Output Power/2(Iq), Stator Voltage/2(Iq)
  [Id] -> Electromagnetic Torque Output Power/1(Id), Stator Voltage/1(Id)
  [Iq] -> Dynamics/2(Iq)
  [Id] -> Dynamics/1(Id)
  Gain2/1 -> [nu]
  Demux/2 -> [Iq]
  Demux/1 -> [Id]
  w/1 -> Gain4/1
  Stator Voltage/1(Ed) -> [Vd]
  Stator Voltage/2(Eq) -> [Vq]
  Dynamics/4(Phi_2q) -> Electromagnetic Torque Output Power/6(Phi_2q), Stator Voltage/6(Phi_2q)
  Dynamics/3(Phi_1d) -> Electromagnetic Torque Output Power/5(Phi_1d), Stator Voltage/5(Phi_1d)
  Dynamics/2(Ed1) -> Electromagnetic Torque Output Power/4(Ed1), Stator Voltage/4(Ed1)
  Dynamics/1(Eq1) -> Electromagnetic Torque Output Power/3(Eq1), Stator Voltage/3(Eq1)
  Temp/1 -> [R_temp_delta]
  Gain1/1 -> Divide/1
  Divide/1 -> [Efd]
  Gain3/1 -> Product/1  "vfd'"
  Product/1 -> Gain1/1, vfd'/1
  [R_temp_delta] -> Divide/2, Product/2
  [R_temp_delta] -> Stator Voltage/8(Temp), Dynamics/4(Temp)

== system Boeing787_NewMission_ElectricalThermal_2013/Electrical/Generation Unit Sync-Sync4/Chopper (Averaged) ==
  vin : Inport
  q : Inport  Port=2
  Temperature : Inport  Port=3
  1/R : Gain  Gain=1/(R_fd_exc*VBFD_exc/IBFD_exc)/100/2*3/100  SaturateOnIntegerOverflow=on  OutDataTypeStr=Inherit: Same as input  ParamDataTypeStr=Inherit: Same as input
  Divide : Product  Inputs=*/
  Dot Product : DotProduct  InputSameDT=on  OutDataTypeStr=Inherit: Inherit via internal rule
  Dot Product1 : DotProduct  InputSameDT=on  OutDataTypeStr=Inherit: Inherit via internal rule
  Gain2 : Gain  Gain=1000*2/3
  Saturation : Saturate  UpperLimit=1  LowerLimit=0
  iout : Outport
  iin : Outport  Port=2
  wires:
  Divide/1 -> Gain2/1
  Temperature/1 -> Divide/2
  1/R/1 -> Divide/1
  Gain2/1 -> iout/1, Dot Product1/1
  vin/1 -> Dot Product/1
  q/1 -> Saturation/1
  Dot Product/1 -> 1/R/1
  Saturation/1 -> Dot Product/2, Dot Product1/2
  Dot Product1/1 -> iin/1

== system Boeing787_NewMission_ElectricalThermal_2013/Electrical/Generation Unit Sync-Sync4/Exciter ==
  note: Dynamic model of P.U. Synchronous Generators v1.0
      | Base frequency is 60 Hz
      | Network transients are omitted
      | by Tutku Buyukdegirmenci
  note: Core Dynaimcs
  note: Outputs
  note: Inputs
  note: 0 axis to be implemented
  idq0 : Inport
  w : Inport  Port=2
  ifd' : Inport  Port=3
  Temp : Inport  Port=4
  Demux : Demux  Outputs=3
  Divide : Product  Inputs=*/
  Dynamics : Subsystem
  Electromagnetic Torque Output Power : Subsystem
  Gain1 : Gain  Gain=Xmd_exc/R_fd_exc/VBFD_exc
  Gain2 : Gain  Gain=1/wB_exc
  Gain3 : Gain  Gain=R_fd_exc*VBFD_exc/IBFD_exc
  Gain4 : Gain  Gain=P_exc/2
  Generator Power Loss : Subsystem
  Mux : Mux  Inputs=3
  Product : Product
  Stator Voltage : Subsystem
  Terminator2 : Terminator
  Terminator3 : Terminator
  Terminator4 : Terminator
  V0 : Constant  Value=0
  p.u. transform currents : Gain  Gain=-1/IBDQ_exc
  p.u. transform torque : Gain  Gain=TB_exc
  p.u. transform voltages : Gain  Gain=VBDQ_exc
  vdq0 : Outport
  Te : Outport  Port=2
  vfd' : Outport  Port=3
  Ploss : Outport  Port=4
  wires:
  [R_temp_delta] -> Divide/2, Product/2
  Product/1 -> Gain1/1, vfd'/1
  Divide/1 -> [Efd]
  Gain1/1 -> Divide/1
  Gain3/1 -> Product/1  "vfd'"
  [R_temp_delta] -> Dynamics/4(Temp), Stator Voltage/8(Temp)
  Temp/1 -> [R_temp_delta]
  Gain4/1 -> Gain2/1
  [Efd] -> Dynamics/3(Efd)
  ifd'/1 -> Gain3/1
  idq0/1 -> p.u. transform currents/1
  p.u. transform voltages/1 -> vdq0/1
  Generator Power Loss/3(PLOSS) -> Terminator4/1, Ploss/1
  Generator Power Loss/2(PM) -> Terminator3/1
  Generator Power Loss/1(PE) -> Terminator2/1
  [Te] -> Generator Power Loss/5(Te)
  [nu] -> Generator Power Loss/6(w/ws)
  [Iq] -> Generator Power Loss/4(Iq)
  [Id] -> Generator Power Loss/3(Id)
  [Vq] -> Generator Power Loss/2(Eq)
  [Vd] -> Generator Power Loss/1(Ed)
  p.u. transform torque/1 -> Te/1
  p.u. transform currents/1 -> Demux/1
  [Te] -> p.u. transform torque/1
  Electromagnetic Torque Output Power/1(TE) -> [Te]
  [nu] -> Stator Voltage/7(w/ws)
  V0/1 -> Mux/3
  [Vq] -> Mux/2
  [Vd] -> Mux/1
  Mux/1 -> p.u. transform voltages/1
  [Iq] -> Electromagnetic Torque Output Power/2(Iq), Stator Voltage/2(Iq)
  [Id] -> Electromagnetic Torque Output Power/1(Id), Stator Voltage/1(Id)
  [Iq] -> Dynamics/2(Iq)
  [Id] -> Dynamics/1(Id)
  Gain2/1 -> [nu]
  Demux/2 -> [Iq]
  Demux/1 -> [Id]
  w/1 -> Gain4/1
  Stator Voltage/1(Ed) -> [Vd]
  Stator Voltage/2(Eq) -> [Vq]
  Dynamics/4(Phi_2q) -> Electromagnetic Torque Output Power/6(Phi_2q), Stator Voltage/6(Phi_2q)
  Dynamics/3(Phi_1d) -> Electromagnetic Torque Output Power/5(Phi_1d), Stator Voltage/5(Phi_1d)
  Dynamics/2(Ed1) -> Electromagnetic Torque Output Power/4(Ed1), Stator Voltage/4(Ed1)
  Dynamics/1(Eq1) -> Electromagnetic Torque Output Power/3(Eq1), Stator Voltage/3(Eq1)

== system Boeing787_NewMission_ElectricalThermal_2013/Electrical/Generation Unit Sync-Sync4/Generator ==
  note: 0 axis to be implemented
  note: Inputs
  note: Outputs
  note: Core Dynaimcs
  note: Dynamic model of P.U. Synchronous Generators v1.0
      | Base frequency is 60 Hz
      | Network transients are omitted
      | by Tutku Buyukdegirmenci
  idq0 : Inport
  w : Inport  Port=2
  ifd' : Inport  Port=3
  Temp : Inport  Port=4
  Demux : Demux  Outputs=3
  Divide : Product  Inputs=*/
  Dynamics : Subsystem
  Electromagnetic Torque Output Power : Subsystem
  Gain1 : Gain  Gain=Xmd/R_fd/VBFD
  Gain2 : Gain  Gain=1/wB
  Gain3 : Gain  Gain=R_fd*VBFD/IBFD
  Gain4 : Gain  Gain=P/2
  Generator Power Loss : Subsystem
  Mux : Mux  Inputs=3
  Product : Product
  Stator Voltage : Subsystem
  Terminator2 : Terminator
  Terminator3 : Terminator
  Terminator4 : Terminator
  V0 : Constant  Value=0
  p.u. transform currents : Gain  Gain=-1/IBDQ
  p.u. transform torque : Gain  Gain=TB
  p.u. transform voltages : Gain  Gain=VBDQ
  vdq0 : Outport
  Te : Outport  Port=2
  vfd' : Outport  Port=3
  Ploss : Outport  Port=4
  wires:
  [R_temp_delta] -> Dynamics/4(Temp), Stator Voltage/8(Temp)
  [R_temp_delta] -> Product/2, Divide/2
  Product/1 -> vfd'/1, Gain1/1
  Gain3/1 -> Product/1  "vfd'"
  Divide/1 -> [Efd]
  Gain1/1 -> Divide/1
  Temp/1 -> [R_temp_delta]
  Dynamics/1(Eq1) -> Stator Voltage/3(Eq1), Electromagnetic Torque Output Power/3(Eq1)
  Dynamics/2(Ed1) -> Stator Voltage/4(Ed1), Electromagnetic Torque Output Power/4(Ed1)
  Dynamics/3(Phi_1d) -> Stator Voltage/5(Phi_1d), Electromagnetic Torque Output Power/5(Phi_1d)
  Dynamics/4(Phi_2q) -> Stator Voltage/6(Phi_2q), Electromagnetic Torque Output Power/6(Phi_2q)
  Stator Voltage/2(Eq) -> [Vq]
  Stator Voltage/1(Ed) -> [Vd]
  w/1 -> Gain4/1
  Demux/1 -> [Id]
  Demux/2 -> [Iq]
  Gain2/1 -> [nu]
  [Id] -> Dynamics/1(Id)
  [Iq] -> Dynamics/2(Iq)
  [Id] -> Stator Voltage/1(Id), Electromagnetic Torque Output Power/1(Id)
  [Iq] -> Stator Voltage/2(Iq), Electromagnetic Torque Output Power/2(Iq)
  Mux/1 -> p.u. transform voltages/1
  [Vd] -> Mux/1
  [Vq] -> Mux/2
  V0/1 -> Mux/3
  [nu] -> Stator Voltage/7(w/ws)
  Electromagnetic Torque Output Power/1(TE) -> [Te]
  [Te] -> p.u. transform torque/1
  p.u. transform currents/1 -> Demux/1
  p.u. transform torque/1 -> Te/1
  [Vd] -> Generator Power Loss/1(Ed)
  [Vq] -> Generator Power Loss/2(Eq)
  [Id] -> Generator Power Loss/3(Id)
  [Iq] -> Generator Power Loss/4(Iq)
  [nu] -> Generator Power Loss/6(w/ws)
  [Te] -> Generator Power Loss/5(Te)
  Generator Power Loss/1(PE) -> Terminator2/1
  Generator Power Loss/2(PM) -> Terminator3/1
  Generator Power Loss/3(PLOSS) -> Terminator4/1, Ploss/1
  p.u. transform voltages/1 -> vdq0/1
  idq0/1 -> p.u. transform currents/1
  ifd'/1 -> Gain3/1
  [Efd] -> Dynamics/3(Efd)
  Gain4/1 -> Gain2/1

== system Boeing787_NewMission_ElectricalThermal_2013/Electrical/Generation Unit Sync-Sync5/Chopper (Averaged) ==
  vin : Inport
  q : Inport  Port=2
  Temperature : Inport  Port=3
  1/R : Gain  Gain=1/(R_fd_exc*VBFD_exc/IBFD_exc)/100/2*3/100  SaturateOnIntegerOverflow=on  OutDataTypeStr=Inherit: Same as input  ParamDataTypeStr=Inherit: Same as input
  Divide : Product  Inputs=*/
  Dot Product : DotProduct  InputSameDT=on  OutDataTypeStr=Inherit: Inherit via internal rule
  Dot Product1 : DotProduct  InputSameDT=on  OutDataTypeStr=Inherit: Inherit via internal rule
  Gain2 : Gain  Gain=1000*2/3
  Saturation : Saturate  UpperLimit=1  LowerLimit=0
  iout : Outport
  iin : Outport  Port=2
  wires:
  Dot Product1/1 -> iin/1
  Saturation/1 -> Dot Product1/2, Dot Product/2
  Dot Product/1 -> 1/R/1
  q/1 -> Saturation/1
  vin/1 -> Dot Product/1
  Gain2/1 -> Dot Product1/1, iout/1
  1/R/1 -> Divide/1
  Temperature/1 -> Divide/2
  Divide/1 -> Gain2/1

== system Boeing787_NewMission_ElectricalThermal_2013/Electrical/Generation Unit Sync-Sync5/Exciter ==
  note: 0 axis to be implemented
  note: Inputs
  note: Outputs
  note: Core Dynaimcs
  note: Dynamic model of P.U. Synchronous Generators v1.0
      | Base frequency is 60 Hz
      | Network transients are omitted
      | by Tutku Buyukdegirmenci
  idq0 : Inport
  w : Inport  Port=2
  ifd' : Inport  Port=3
  Temp : Inport  Port=4
  Demux : Demux  Outputs=3
  Divide : Product  Inputs=*/
  Dynamics : Subsystem
  Electromagnetic Torque Output Power : Subsystem
  Gain1 : Gain  Gain=Xmd_exc/R_fd_exc/VBFD_exc
  Gain2 : Gain  Gain=1/wB_exc
  Gain3 : Gain  Gain=R_fd_exc*VBFD_exc/IBFD_exc
  Gain4 : Gain  Gain=P_exc/2
  Generator Power Loss : Subsystem
  Mux : Mux  Inputs=3
  Product : Product
  Stator Voltage : Subsystem
  Terminator2 : Terminator
  Terminator3 : Terminator
  Terminator4 : Terminator
  V0 : Constant  Value=0
  p.u. transform currents : Gain  Gain=-1/IBDQ_exc
  p.u. transform torque : Gain  Gain=TB_exc
  p.u. transform voltages : Gain  Gain=VBDQ_exc
  vdq0 : Outport
  Te : Outport  Port=2
  vfd' : Outport  Port=3
  Ploss : Outport  Port=4
  wires:
  Dynamics/1(Eq1) -> Stator Voltage/3(Eq1), Electromagnetic Torque Output Power/3(Eq1)
  Dynamics/2(Ed1) -> Stator Voltage/4(Ed1), Electromagnetic Torque Output Power/4(Ed1)
  Dynamics/3(Phi_1d) -> Stator Voltage/5(Phi_1d), Electromagnetic Torque Output Power/5(Phi_1d)
  Dynamics/4(Phi_2q) -> Stator Voltage/6(Phi_2q), Electromagnetic Torque Output Power/6(Phi_2q)
  Stator Voltage/2(Eq) -> [Vq]
  Stator Voltage/1(Ed) -> [Vd]
  w/1 -> Gain4/1
  Demux/1 -> [Id]
  Demux/2 -> [Iq]
  Gain2/1 -> [nu]
  [Id] -> Dynamics/1(Id)
  [Iq] -> Dynamics/2(Iq)
  [Id] -> Stator Voltage/1(Id), Electromagnetic Torque Output Power/1(Id)
  [Iq] -> Stator Voltage/2(Iq), Electromagnetic Torque Output Power/2(Iq)
  Mux/1 -> p.u. transform voltages/1
  [Vd] -> Mux/1
  [Vq] -> Mux/2
  V0/1 -> Mux/3
  [nu] -> Stator Voltage/7(w/ws)
  Electromagnetic Torque Output Power/1(TE) -> [Te]
  [Te] -> p.u. transform torque/1
  p.u. transform currents/1 -> Demux/1
  p.u. transform torque/1 -> Te/1
  [Vd] -> Generator Power Loss/1(Ed)
  [Vq] -> Generator Power Loss/2(Eq)
  [Id] -> Generator Power Loss/3(Id)
  [Iq] -> Generator Power Loss/4(Iq)
  [nu] -> Generator Power Loss/6(w/ws)
  [Te] -> Generator Power Loss/5(Te)
  Generator Power Loss/1(PE) -> Terminator2/1
  Generator Power Loss/2(PM) -> Terminator3/1
  Generator Power Loss/3(PLOSS) -> Ploss/1, Terminator4/1
  p.u. transform voltages/1 -> vdq0/1
  idq0/1 -> p.u. transform currents/1
  ifd'/1 -> Gain3/1
  [Efd] -> Dynamics/3(Efd)
  Gain4/1 -> Gain2/1
  Temp/1 -> [R_temp_delta]
  [R_temp_delta] -> Stator Voltage/8(Temp), Dynamics/4(Temp)
  Gain3/1 -> Product/1  "vfd'"
  Gain1/1 -> Divide/1
  Divide/1 -> [Efd]
  Product/1 -> vfd'/1, Gain1/1
  [R_temp_delta] -> Product/2, Divide/2

== system Boeing787_NewMission_ElectricalThermal_2013/Electrical/Generation Unit Sync-Sync5/Generator ==
  note: Dynamic model of P.U. Synchronous Generators v1.0
      | Base frequency is 60 Hz
      | Network transients are omitted
      | by Tutku Buyukdegirmenci
  note: Core Dynaimcs
  note: Outputs
  note: Inputs
  note: 0 axis to be implemented
  idq0 : Inport
  w : Inport  Port=2
  ifd' : Inport  Port=3
  Temp : Inport  Port=4
  Demux : Demux  Outputs=3
  Divide : Product  Inputs=*/
  Dynamics : Subsystem
  Electromagnetic Torque Output Power : Subsystem
  Gain1 : Gain  Gain=Xmd/R_fd/VBFD
  Gain2 : Gain  Gain=1/wB
  Gain3 : Gain  Gain=R_fd*VBFD/IBFD
  Gain4 : Gain  Gain=P/2
  Generator Power Loss : Subsystem
  Mux : Mux  Inputs=3
  Product : Product
  Stator Voltage : Subsystem
  Terminator2 : Terminator
  Terminator3 : Terminator
  Terminator4 : Terminator
  V0 : Constant  Value=0
  p.u. transform currents : Gain  Gain=-1/IBDQ
  p.u. transform torque : Gain  Gain=TB
  p.u. transform voltages : Gain  Gain=VBDQ
  vdq0 : Outport
  Te : Outport  Port=2
  vfd' : Outport  Port=3
  Ploss : Outport  Port=4
  wires:
  Gain4/1 -> Gain2/1
  [Efd] -> Dynamics/3(Efd)
  ifd'/1 -> Gain3/1
  idq0/1 -> p.u. transform currents/1
  p.u. transform voltages/1 -> vdq0/1
  Generator Power Loss/3(PLOSS) -> Ploss/1, Terminator4/1
  Generator Power Loss/2(PM) -> Terminator3/1
  Generator Power Loss/1(PE) -> Terminator2/1
  [Te] -> Generator Power Loss/5(Te)
  [nu] -> Generator Power Loss/6(w/ws)
  [Iq] -> Generator Power Loss/4(Iq)
  [Id] -> Generator Power Loss/3(Id)
  [Vq] -> Generator Power Loss/2(Eq)
  [Vd] -> Generator Power Loss/1(Ed)
  p.u. transform torque/1 -> Te/1
  p.u. transform currents/1 -> Demux/1
  [Te] -> p.u. transform torque/1
  Electromagnetic Torque Output Power/1(TE) -> [Te]
  [nu] -> Stator Voltage/7(w/ws)
  V0/1 -> Mux/3
  [Vq] -> Mux/2
  [Vd] -> Mux/1
  Mux/1 -> p.u. transform voltages/1
  [Iq] -> Electromagnetic Torque Output Power/2(Iq), Stator Voltage/2(Iq)
  [Id] -> Electromagnetic Torque Output Power/1(Id), Stator Voltage/1(Id)
  [Iq] -> Dynamics/2(Iq)
  [Id] -> Dynamics/1(Id)
  Gain2/1 -> [nu]
  Demux/2 -> [Iq]
  Demux/1 -> [Id]
  w/1 -> Gain4/1
  Stator Voltage/1(Ed) -> [Vd]
  Stator Voltage/2(Eq) -> [Vq]
  Dynamics/4(Phi_2q) -> Electromagnetic Torque Output Power/6(Phi_2q), Stator Voltage/6(Phi_2q)
  Dynamics/3(Phi_1d) -> Electromagnetic Torque Output Power/5(Phi_1d), Stator Voltage/5(Phi_1d)
  Dynamics/2(Ed1) -> Electromagnetic Torque Output Power/4(Ed1), Stator Voltage/4(Ed1)
  Dynamics/1(Eq1) -> Electromagnetic Torque Output Power/3(Eq1), Stator Voltage/3(Eq1)
  Temp/1 -> [R_temp_delta]
  Gain1/1 -> Divide/1
  Divide/1 -> [Efd]
  Gain3/1 -> Product/1  "vfd'"
  Product/1 -> Gain1/1, vfd'/1
  [R_temp_delta] -> Divide/2, Product/2
  [R_temp_delta] -> Stator Voltage/8(Temp), Dynamics/4(Temp)

== system Boeing787_NewMission_ElectricalThermal_2013/Electrical/Thermal Interface/Battery Thermal Model ==
  Ploss : Inport
  Liquid Coolant Temp : Inport  Port=2
  Air Temp : Inport  Port=3
  coolant mdot : Inport  Port=4
  Integrator : Integrator  InitialCondition=20
  MATLAB Function : MATLAB Function  TreatAsAtomicUnit=on
      settings: PermitHierarchicalResolution=ParametersOnly
  T_Batt : Outport
  wires:
  Ploss/1 -> MATLAB Function/1(Ploss)
  Liquid Coolant Temp/1 -> MATLAB Function/2(Tf)
  MATLAB Function/1(Tdot) -> Integrator/1
  Integrator/1 -> MATLAB Function/5(Tgen), T_Batt/1
  coolant mdot/1 -> MATLAB Function/4(mdot_f)
  Air Temp/1 -> MATLAB Function/3(Ta)

== system Boeing787_NewMission_ElectricalThermal_2013/Electrical/Thermal Interface/Generator 1 Thermal Model ==
  Ploss : Inport
  Liquid Coolant Temp : Inport  Port=2
  Air Temp : Inport  Port=3
  coolant mdot : Inport  Port=4
  Integrator : Integrator  InitialCondition=20
  MATLAB Function : MATLAB Function  TreatAsAtomicUnit=on
      settings: PermitHierarchicalResolution=ParametersOnly
  T_gen : Outport
  wires:
  Ploss/1 -> MATLAB Function/1(Ploss)
  Liquid Coolant Temp/1 -> MATLAB Function/2(Tf)
  MATLAB Function/1(Tdot) -> Integrator/1
  Integrator/1 -> T_gen/1, MATLAB Function/5(Tgen)
  coolant mdot/1 -> MATLAB Function/4(mdot_f)
  Air Temp/1 -> MATLAB Function/3(Ta)

== system Boeing787_NewMission_ElectricalThermal_2013/Electrical/Thermal Interface/Generator 2 Thermal Model ==
  Ploss : Inport
  Liquid Coolant Temp : Inport  Port=2
  Air Temp : Inport  Port=3
  coolant mdot : Inport  Port=4
  Integrator : Integrator  InitialCondition=20
  MATLAB Function : MATLAB Function  TreatAsAtomicUnit=on
      settings: PermitHierarchicalResolution=ParametersOnly
  T_gen : Outport
  wires:
  Air Temp/1 -> MATLAB Function/3(Ta)
  coolant mdot/1 -> MATLAB Function/4(mdot_f)
  Integrator/1 -> T_gen/1, MATLAB Function/5(Tgen)
  MATLAB Function/1(Tdot) -> Integrator/1
  Liquid Coolant Temp/1 -> MATLAB Function/2(Tf)
  Ploss/1 -> MATLAB Function/1(Ploss)

== system Boeing787_NewMission_ElectricalThermal_2013/Electrical/Thermal Interface/Generator 3 Thermal Model ==
  Ploss : Inport
  Liquid Coolant Temp : Inport  Port=2
  Air Temp : Inport  Port=3
  coolant mdot : Inport  Port=4
  Integrator : Integrator  InitialCondition=20
  MATLAB Function : MATLAB Function  TreatAsAtomicUnit=on
      settings: PermitHierarchicalResolution=ParametersOnly
  T_gen : Outport
  wires:
  Ploss/1 -> MATLAB Function/1(Ploss)
  Liquid Coolant Temp/1 -> MATLAB Function/2(Tf)
  MATLAB Function/1(Tdot) -> Integrator/1
  Integrator/1 -> MATLAB Function/5(Tgen), T_gen/1
  coolant mdot/1 -> MATLAB Function/4(mdot_f)
  Air Temp/1 -> MATLAB Function/3(Ta)
